simulink library "sm_rollerV_lib_terrain_contact_belem"  (R2026a)
settings: Solver=VariableStepAuto
undefined symbols (not defined in the file): Excv, L1, L2, L3, L4, L5, L6, L7, L8, L9, S1, S2, Scene, X, Y, Z
libraries: sm_lib x16, $bdroot x14, nesl_utility x10, sm_trackV_lib_terrain_contact_elem x6
Description:
  | Copyright 2024-2026 The MathWorks, Inc.
settings Model: Creator=smiller  LastModifiedBy=smiller

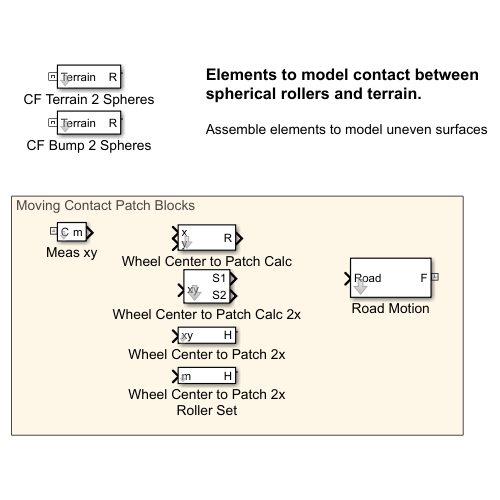
[thumbnail: Simulink's stored preview of the top-level diagram]
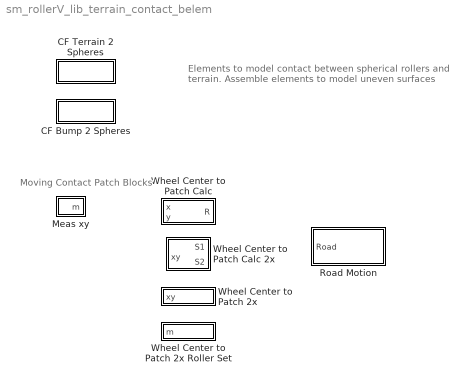
== system sm_rollerV_lib_terrain_contact_belem ==
  note: Moving Contact Patch Blocks
  note: Elements to model contact between
      | spherical rollers and terrain.
      |
      | Assemble elements to model uneven surfaces
  CF Bump 2 Spheres : Subsystem  mask(Contact Force, Two Spheres to Bump){K_BrickBump=Scene.Contact.BrickBump.K, B_BrickBump=Scene.Contact.BrickBump.B, TW_BrickBump=Scene.Contact.BrickBump.TW, CoefficientOfDynamicFriction=Scene.Contact.Terrain.mud, CoefficientOfStaticFriction=Scene.Contact.Terrain.mus, FrictionalCriticalVelocity=Scene.Contact.Terrain.CV}
      mask prompts: K_BrickBump "Normal Stiffness (N/m)"; B_BrickBump "Normal Damping (N/(m/s))"; TW_BrickBump "Normal Transition Width (m)"; CoefficientOfDynamicFriction "Coefficient of Dynamic Friction"; CoefficientOfStaticFriction "Coefficient of Static Friction"; FrictionalCriticalVelocity "Critical Velocity (m/s)"
      mask help: Models contact force between two spheres and a bump.
      mask TypeOptions K_BrickBump: CF Bump Roller Sphere 1 /NormalStiffness | CF Bump Roller Sphere 2/NormalStiffness
      mask TypeOptions B_BrickBump: CF Bump Roller Sphere 1 /NormalDamping | CF Bump Roller Sphere 2/NormalDamping
      mask TypeOptions TW_BrickBump: CF Bump Roller Sphere 1 /NormalTransitionRegionWidth | CF Bump Roller Sphere 2/NormalTransitionRegionWidth
      mask TypeOptions CoefficientOfDynamicFriction: CF Bump Roller Sphere 1 /CoefficientOfDynamicFriction | CF Bump Roller Sphere 2/CoefficientOfDynamicFriction
      mask TypeOptions CoefficientOfStaticFriction: CF Bump Roller Sphere 1 /CoefficientOfStaticFriction | CF Bump Roller Sphere 2/CoefficientOfStaticFriction
      mask TypeOptions FrictionalCriticalVelocity: CF Bump Roller Sphere 1 /FrictionalCriticalVelocity | CF Bump Roller Sphere 2/FrictionalCriticalVelocity
  CF Terrain 2 Spheres : Subsystem  mask(Contact Force, Two Spheres to Ground){NormalStiffness=Scene.Contact.Spheres.Terrain.K, NormalDamping=Scene.Contact.Spheres.Terrain.B, NormalTransitionRegionWidth=Scene.Contact.Spheres.Terrain.TW, CoefficientOfDynamicFriction=Scene.Contact.Spheres.Terrain.mud, CoefficientOfStaticFriction=Scene.Contact.Spheres.Terrain.mus, FrictionalCriticalVelocity=Scene.Contact.Spheres.Terrain.CV}
      mask prompts: NormalStiffness "Normal Stiffness (N/m)"; NormalDamping "Normal Damping (N/(m/s))"; NormalTransitionRegionWidth "Normal Transition Width (m)"; CoefficientOfDynamicFriction "Coefficient of Dynamic Friction"; CoefficientOfStaticFriction "Coefficient of Static Friction"; FrictionalCriticalVelocity "Critical Velocity (m/s)"
      mask help: Models contact force between two spheres and the ground.
      mask TypeOptions NormalStiffness: CF Roller Sphere Terrain 1/NormalStiffness | CF Roller Sphere Terrain 2/NormalStiffness
      mask TypeOptions NormalDamping: CF Roller Sphere Terrain 1/NormalDamping | CF Roller Sphere Terrain 2/NormalDamping
      mask TypeOptions NormalTransitionRegionWidth: CF Roller Sphere Terrain 1/NormalTransitionRegionWidth | CF Roller Sphere Terrain 2/NormalTransitionRegionWidth
      mask TypeOptions CoefficientOfDynamicFriction: CF Roller Sphere Terrain 1/CoefficientOfDynamicFriction | CF Roller Sphere Terrain 2/CoefficientOfDynamicFriction
      mask TypeOptions CoefficientOfStaticFriction: CF Roller Sphere Terrain 1/CoefficientOfStaticFriction | CF Roller Sphere Terrain 2/CoefficientOfStaticFriction
      mask TypeOptions FrictionalCriticalVelocity: CF Roller Sphere Terrain 1/FrictionalCriticalVelocity | CF Roller Sphere Terrain 2/FrictionalCriticalVelocity
  Meas xy : Subsystem  mask(Measure Cartesian Location of two frames){whl_offset=Excv.Shoe.w}
      mask prompts: whl_offset "Frame Offset"
      mask help: Measure position of two frames. Frames are separated by a distance along their common z-axis.
  Road Motion : Subsystem  mask(Position Infinite Plane){}
      mask help: Positions and orients Infinite Plane based on input signal. Abstract method of modeling objects contacting uneven terrain.
  Wheel Center to Patch 2x : Subsystem  mask(Wheel Center to Patch Height and Pitch, Infinite Planes){road_pz_x=Scene.Plateau.Road.pzLUT.px, road_pz_z=Scene.Plateau.Road.pzLUT.pz(:,1), road_qy_x=Scene.Plateau.Road.qyLUT.px, road_qy_qy=Scene.Plateau.Road.qyLUT.qy(:,1), tfilter=0.01, patch_clr=[0.5 0.5 0.5], patch_opc=0.25, patch_x=1, patch_y=1, NormalStiffness=Scene.Contact.Terrain.K, NormalDamping=Scene.Contact.Terrain.B, NormalTransitionRegionWidth=Scene.Contact.Terrain.TW, CoefficientOfDynamicFriction=Scene.Contact.Terrain.mud, CoefficientOfStaticFriction=Scene.Contact.Terrain.mus, FrictionalCriticalVelocity=Scene.Contact.Terrain.CV}
      mask prompts: road_pz_x "Road Distances (m)"; road_pz_z "Road Heights (m)"; road_qy_x "Road Distances(m)"; road_qy_qy "Road Pitch (m)"; tfilter "Filter Constant (seconds)"; patch_clr "Color [R G B] (0-1)"; patch_opc "Opacity (0-1)"; patch_x "Patch Length x (m)"; patch_y "Patch Length y (m)"; NormalStiffness "Normal Stiffness (N/m)"; NormalDamping "Normal Damping (N/(m/s))"; NormalTransitionRegionWidth "Normal Transition Width (m)"; CoefficientOfDynamicFriction "Coefficient of Dynamic Friction"; CoefficientOfStaticFriction "Coefficient of Static Friction"; FrictionalCriticalVelocity "Critical Velocity (m/s)"
      mask help: Find contact patch height and pitch using a lookup table, where the inputs are the x-y location of two frames. The output is a Simscape Bus with the geometry ports for Infinite Planes positioned and pitched for the two input frame locations.
      mask TypeOptions road_pz_x:
      | Wheel Center
      | to Patch/road_pz_x
      mask TypeOptions road_pz_z:
      | Wheel Center
      | to Patch/road_pz_z
      mask TypeOptions road_qy_x:
      | Wheel Center
      | to Patch/road_qy_x
      mask TypeOptions road_qy_qy:
      | Wheel Center
      | to Patch/road_qy_qy
      mask TypeOptions tfilter:
      | Wheel Center
      | to Patch/tfilter
      mask TypeOptions patch_clr: Infinite Plane1/GraphicDiffuseColor | Infinite Plane2/GraphicDiffuseColor
      mask TypeOptions patch_opc: Infinite Plane1/GraphicOpacity | Infinite Plane2/GraphicOpacity
      mask TypeOptions patch_x: Infinite Plane1/GraphicPlaneWidth | Infinite Plane2/GraphicPlaneWidth
      mask TypeOptions patch_y: Infinite Plane1/GraphicPlaneHeight | Infinite Plane2/GraphicPlaneHeight
      mask TypeOptions NormalStiffness: CF Track Terrain1/NormalStiffness | CF Track Terrain2/NormalStiffness
      mask TypeOptions NormalDamping: CF Track Terrain1/NormalDamping | CF Track Terrain2/NormalDamping
      mask TypeOptions NormalTransitionRegionWidth: CF Track Terrain1/NormalTransitionRegionWidth | CF Track Terrain2/NormalTransitionRegionWidth
      mask TypeOptions CoefficientOfDynamicFriction: CF Track Terrain1/CoefficientOfDynamicFriction | CF Track Terrain2/CoefficientOfDynamicFriction
      mask TypeOptions CoefficientOfStaticFriction: CF Track Terrain1/CoefficientOfStaticFriction | CF Track Terrain2/CoefficientOfStaticFriction
      mask TypeOptions FrictionalCriticalVelocity: CF Track Terrain1/FrictionalCriticalVelocity | CF Track Terrain2/FrictionalCriticalVelocity
      mask DialogControl cont_surface Prompt: Surface
      mask DialogControl cont_patchvis Prompt: Patch Visual
      mask DialogControl cont_contact Prompt: Contact
  Wheel Center to Patch 2x Roller Set : Subsystem  mask(Wheel Center to Patch Height and Pitch, All Rollers){road_pz_x=Scene.Plateau.Road.pzLUT.px, road_pz_z=Scene.Plateau.Road.pzLUT.pz(:,1), road_qy_x=Scene.Plateau.Road.qyLUT.px, road_qy_qy=Scene.Plateau.Road.qyLUT.qy(:,1), tfilter=0.01, NormalStiffness=Scene.Contact.Terrain.K, NormalDamping=Scene.Contact.Terrain.B, NormalTransitionRegionWidth=Scene.Contact.Terrain.TW, CoefficientOfDynamicFriction=Scene.Contact.Terrain.mud, CoefficientOfStaticFriction=Scene.Contact.Terrain.mus, FrictionalCriticalVelocity=Scene.Contact.Terrain.CV, patch_x=1, patch_y=1, patch_clr=[0.5 0.5 0.5], patch_opc=0.25}
      mask prompts: road_pz_x "Road Distances (m)"; road_pz_z "Road Heights (m)"; road_qy_x "Road Distances(m)"; road_qy_qy "Road Pitch (m)"; tfilter "Filter Constant (seconds)"; NormalStiffness "Normal Stiffness (N/m)"; NormalDamping "Normal Damping (N/(m/s))"; NormalTransitionRegionWidth "Normal Transition Width (m)"; CoefficientOfDynamicFriction "Coefficient of Dynamic Friction"; CoefficientOfStaticFriction "Coefficient of Static Friction"; FrictionalCriticalVelocity "Critical Velocity (m/s)"; patch_x "Patch Length x (m)"; patch_y "Patch Length y (m)"; patch_clr "Color [R G B] (0-1)"; patch_opc "Opacity (0-1)"
      mask help: Find contact patch height and pitch using a lookup table, where the inputs are the x-y location of two frames. The output is a Simscape Bus with the geometry ports for Infinite Planes positioned and pitched for all input frame locations.
      mask TypeOptions road_pz_x: Wheel Center to Patch Contact 1/road_pz_x | Wheel Center to Patch Contact 2/road_pz_x | Wheel Center to Patch Contact 3/road_pz_x | Wheel Center to Patch Contact 4/road_pz_x | Wheel Center to Patch Contact 5/road_pz_x | Wheel Center to Patch Contact 6/road_pz_x | Wheel Center to Patch Contact 7/road_pz_x | Wheel Center to Patch Contact 8/road_pz_x | Wheel Center to Patch Contact 9/road_pz_x
      mask TypeOptions road_pz_z: Wheel Center to Patch Contact 1/road_pz_z | Wheel Center to Patch Contact 2/road_pz_z | Wheel Center to Patch Contact 3/road_pz_z | Wheel Center to Patch Contact 4/road_pz_z | Wheel Center to Patch Contact 5/road_pz_z | Wheel Center to Patch Contact 6/road_pz_z | Wheel Center to Patch Contact 7/road_pz_z | Wheel Center to Patch Contact 8/road_pz_z | Wheel Center to Patch Contact 9/road_pz_z
      mask TypeOptions road_qy_x: Wheel Center to Patch Contact 1/road_qy_x | Wheel Center to Patch Contact 2/road_qy_x | Wheel Center to Patch Contact 3/road_qy_x | Wheel Center to Patch Contact 4/road_qy_x | Wheel Center to Patch Contact 5/road_qy_x | Wheel Center to Patch Contact 6/road_qy_x | Wheel Center to Patch Contact 7/road_qy_x | Wheel Center to Patch Contact 8/road_qy_x | Wheel Center to Patch Contact 9/road_qy_x
      mask TypeOptions road_qy_qy: Wheel Center to Patch Contact 1/road_qy_qy | Wheel Center to Patch Contact 2/road_qy_qy | Wheel Center to Patch Contact 3/road_qy_qy | Wheel Center to Patch Contact 4/road_qy_qy | Wheel Center to Patch Contact 5/road_qy_qy | Wheel Center to Patch Contact 6/road_qy_qy | Wheel Center to Patch Contact 7/road_qy_qy | Wheel Center to Patch Contact 8/road_qy_qy | Wheel Center to Patch Contact 9/road_qy_qy
      mask TypeOptions tfilter: Wheel Center to Patch Contact 1/tfilter | Wheel Center to Patch Contact 2/tfilter | Wheel Center to Patch Contact 3/tfilter | Wheel Center to Patch Contact 4/tfilter | Wheel Center to Patch Contact 5/tfilter | Wheel Center to Patch Contact 6/tfilter | Wheel Center to Patch Contact 7/tfilter | Wheel Center to Patch Contact 8/tfilter | Wheel Center to Patch Contact 9/tfilter
      mask TypeOptions NormalStiffness: Wheel Center to Patch Contact 1/NormalStiffness | Wheel Center to Patch Contact 2/NormalStiffness | Wheel Center to Patch Contact 3/NormalStiffness | Wheel Center to Patch Contact 4/NormalStiffness | Wheel Center to Patch Contact 5/NormalStiffness | Wheel Center to Patch Contact 6/NormalStiffness | Wheel Center to Patch Contact 7/NormalStiffness | Wheel Center to Patch Contact 8/NormalStiffness | Wheel Center to Patch Contact 9/NormalStiffness
      mask TypeOptions NormalDamping: Wheel Center to Patch Contact 1/NormalDamping | Wheel Center to Patch Contact 2/NormalDamping | Wheel Center to Patch Contact 3/NormalDamping | Wheel Center to Patch Contact 4/NormalDamping | Wheel Center to Patch Contact 5/NormalDamping | Wheel Center to Patch Contact 6/NormalDamping | Wheel Center to Patch Contact 7/NormalDamping | Wheel Center to Patch Contact 8/NormalDamping | Wheel Center to Patch Contact 9/NormalDamping
      mask TypeOptions NormalTransitionRegionWidth: Wheel Center to Patch Contact 1/NormalTransitionRegionWidth | Wheel Center to Patch Contact 2/NormalTransitionRegionWidth | Wheel Center to Patch Contact 3/NormalTransitionRegionWidth | Wheel Center to Patch Contact 4/NormalTransitionRegionWidth | Wheel Center to Patch Contact 5/NormalTransitionRegionWidth | Wheel Center to Patch Contact 6/NormalTransitionRegionWidth | Wheel Center to Patch Contact 7/NormalTransitionRegionWidth | Wheel Center to Patch Contact 8/NormalTransitionRegionWidth | Wheel Center to Patch Contact 9/NormalTransitionRegionWidth
      mask TypeOptions CoefficientOfDynamicFriction: Wheel Center to Patch Contact 1/CoefficientOfDynamicFriction | Wheel Center to Patch Contact 2/CoefficientOfDynamicFriction | Wheel Center to Patch Contact 3/CoefficientOfDynamicFriction | Wheel Center to Patch Contact 4/CoefficientOfDynamicFriction | Wheel Center to Patch Contact 5/CoefficientOfDynamicFriction | Wheel Center to Patch Contact 6/CoefficientOfDynamicFriction | Wheel Center to Patch Contact 7/CoefficientOfDynamicFriction | Wheel Center to Patch Contact 8/CoefficientOfDynamicFriction | Wheel Center to Patch Contact 9/CoefficientOfDynamicFriction
      mask TypeOptions CoefficientOfStaticFriction: Wheel Center to Patch Contact 1/CoefficientOfStaticFriction | Wheel Center to Patch Contact 2/CoefficientOfStaticFriction | Wheel Center to Patch Contact 3/CoefficientOfStaticFriction | Wheel Center to Patch Contact 4/CoefficientOfStaticFriction | Wheel Center to Patch Contact 5/CoefficientOfStaticFriction | Wheel Center to Patch Contact 6/CoefficientOfStaticFriction | Wheel Center to Patch Contact 7/CoefficientOfStaticFriction | Wheel Center to Patch Contact 8/CoefficientOfStaticFriction | Wheel Center to Patch Contact 9/CoefficientOfStaticFriction
      mask TypeOptions FrictionalCriticalVelocity: Wheel Center to Patch Contact 1/FrictionalCriticalVelocity | Wheel Center to Patch Contact 2/FrictionalCriticalVelocity | Wheel Center to Patch Contact 3/FrictionalCriticalVelocity | Wheel Center to Patch Contact 4/FrictionalCriticalVelocity | Wheel Center to Patch Contact 5/FrictionalCriticalVelocity | Wheel Center to Patch Contact 6/FrictionalCriticalVelocity | Wheel Center to Patch Contact 7/FrictionalCriticalVelocity | Wheel Center to Patch Contact 8/FrictionalCriticalVelocity | Wheel Center to Patch Contact 9/FrictionalCriticalVelocity
      mask TypeOptions patch_x: Wheel Center to Patch Contact 1/patch_x | Wheel Center to Patch Contact 2/patch_x | Wheel Center to Patch Contact 3/patch_x | Wheel Center to Patch Contact 4/patch_x | Wheel Center to Patch Contact 5/patch_x | Wheel Center to Patch Contact 6/patch_x | Wheel Center to Patch Contact 7/patch_x | Wheel Center to Patch Contact 8/patch_x | Wheel Center to Patch Contact 9/patch_x
      mask TypeOptions patch_y: Wheel Center to Patch Contact 1/patch_y | Wheel Center to Patch Contact 2/patch_y | Wheel Center to Patch Contact 3/patch_y | Wheel Center to Patch Contact 4/patch_y | Wheel Center to Patch Contact 5/patch_y | Wheel Center to Patch Contact 6/patch_y | Wheel Center to Patch Contact 7/patch_y | Wheel Center to Patch Contact 8/patch_y | Wheel Center to Patch Contact 9/patch_y
      mask TypeOptions patch_clr: Wheel Center to Patch Contact 1/patch_clr | Wheel Center to Patch Contact 2/patch_clr | Wheel Center to Patch Contact 3/patch_clr | Wheel Center to Patch Contact 4/patch_clr | Wheel Center to Patch Contact 5/patch_clr | Wheel Center to Patch Contact 6/patch_clr | Wheel Center to Patch Contact 7/patch_clr | Wheel Center to Patch Contact 8/patch_clr | Wheel Center to Patch Contact 9/patch_clr
      mask TypeOptions patch_opc: Wheel Center to Patch Contact 1/patch_opc | Wheel Center to Patch Contact 2/patch_opc | Wheel Center to Patch Contact 3/patch_opc | Wheel Center to Patch Contact 4/patch_opc | Wheel Center to Patch Contact 5/patch_opc | Wheel Center to Patch Contact 6/patch_opc | Wheel Center to Patch Contact 7/patch_opc | Wheel Center to Patch Contact 8/patch_opc | Wheel Center to Patch Contact 9/patch_opc
      mask DialogControl cont_surface Prompt: Surface
      mask DialogControl cont_surfHeight Prompt: Height
      mask DialogControl cont_surfPitch Prompt: Pitch
      mask DialogControl cont_contact Prompt: Contact
      mask DialogControl cont_patchvis Prompt: Patch Visual
  Wheel Center to Patch Calc : Subsystem  mask(Wheel Center to Patch Height and Pitch){road_pz_x=Scene.Plateau.Road.pzLUT.px, road_pz_z=Scene.Plateau.Road.pzLUT.pz(:,1), road_qy_x=Scene.Plateau.Road.qyLUT.px, road_qy_qy=Scene.Plateau.Road.qyLUT.qy(:,1)}
      mask prompts: road_pz_x "Road Distances (m)"; road_pz_z "Road Heights (m)"; road_qy_x "Road Distances(m)"; road_qy_qy "Road Pitch (m)"
      mask help: Find contact patch height and pitch using a lookup table, where the inputs are the x-y location of the frame.
      mask DialogControl cont_roadpz Prompt: Road Height
      mask DialogControl cont_roadqy Prompt: Road Pitch
  Wheel Center to Patch Calc 2x : Subsystem  mask(Wheel Center to Patch Height and Pitch, Two Frames){road_pz_x=Scene.Plateau.Road.pzLUT.px, road_pz_z=Scene.Plateau.Road.pzLUT.pz(:,1), road_qy_x=Scene.Plateau.Road.qyLUT.px, road_qy_qy=Scene.Plateau.Road.qyLUT.qy(:,1), tfilter=0.01}
      mask prompts: road_pz_x "Road Distances (m)"; road_pz_z "Road Heights (m)"; road_qy_x "Road Distances(m)"; road_qy_qy "Road Pitch (m)"; tfilter "Filter Constant (seconds)"
      mask help: Find contact patch height and pitch using a lookup table, where the inputs are the x-y location of two frames.
      mask TypeOptions road_pz_x: Wheel Center to Patch1/road_pz_x | Wheel Center to Patch2/road_pz_x
      mask TypeOptions road_pz_z: Wheel Center to Patch1/road_pz_z | Wheel Center to Patch2/road_pz_z
      mask TypeOptions road_qy_x: Wheel Center to Patch1/road_qy_x | Wheel Center to Patch2/road_qy_x
      mask TypeOptions road_qy_qy: Wheel Center to Patch1/road_qy_qy | Wheel Center to Patch2/road_qy_qy

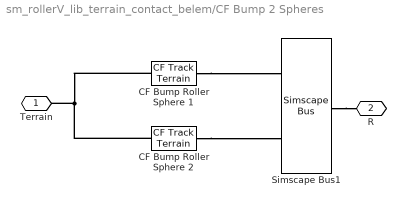
== system sm_rollerV_lib_terrain_contact_belem/CF Bump 2 Spheres ==
  "CF Bump Roller Sphere 1 " : sm_trackV_lib_terrain_contact_elem/CF Track Terrain  NormalStiffness=K_BrickBump  NormalDamping=B_BrickBump  NormalTransitionRegionWidth=TW_BrickBump  CoefficientOfDynamicFriction=CoefficientOfDynamicFriction  CoefficientOfStaticFriction=CoefficientOfStaticFriction  FrictionalCriticalVelocity=FrictionalCriticalVelocity
  CF Bump Roller Sphere 2 : sm_trackV_lib_terrain_contact_elem/CF Track Terrain  NormalStiffness=K_BrickBump  NormalDamping=B_BrickBump  NormalTransitionRegionWidth=TW_BrickBump  CoefficientOfDynamicFriction=CoefficientOfDynamicFriction  CoefficientOfStaticFriction=CoefficientOfStaticFriction  FrictionalCriticalVelocity=FrictionalCriticalVelocity
  Simscape Bus1 : SimscapeBus  HierarchyStrings=S1;S2
  Terrain : PMIOPort  Side=Left
  R : PMIOPort  Port=2  Side=Right
  connections:
  "CF Bump Roller Sphere 1 "/RConn1 -- Simscape Bus1/LConn1
  "CF Bump Roller Sphere 1 "/LConn1 -- CF Bump Roller Sphere 2/LConn1 -- Terrain/RConn1
  CF Bump Roller Sphere 2/RConn1 -- Simscape Bus1/LConn2
  Simscape Bus1/RConn1 -- R/RConn1

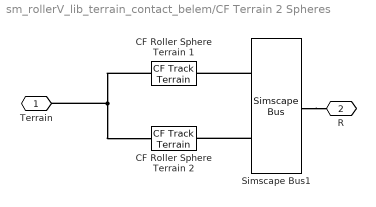
== system sm_rollerV_lib_terrain_contact_belem/CF Terrain 2 Spheres ==
  CF Roller Sphere Terrain 1 : sm_trackV_lib_terrain_contact_elem/CF Track Terrain  NormalStiffness=NormalStiffness  NormalDamping=NormalDamping  NormalTransitionRegionWidth=NormalTransitionRegionWidth  CoefficientOfDynamicFriction=CoefficientOfDynamicFriction  CoefficientOfStaticFriction=CoefficientOfStaticFriction  FrictionalCriticalVelocity=FrictionalCriticalVelocity
  CF Roller Sphere Terrain 2 : sm_trackV_lib_terrain_contact_elem/CF Track Terrain  NormalStiffness=NormalStiffness  NormalDamping=NormalDamping  NormalTransitionRegionWidth=NormalTransitionRegionWidth  CoefficientOfDynamicFriction=CoefficientOfDynamicFriction  CoefficientOfStaticFriction=CoefficientOfStaticFriction  FrictionalCriticalVelocity=FrictionalCriticalVelocity
  Simscape Bus1 : SimscapeBus  HierarchyStrings=S1;S2
  Terrain : PMIOPort  Side=Left
  R : PMIOPort  Port=2  Side=Right
  connections:
  Simscape Bus1/RConn1 -- R/RConn1
  Simscape Bus1/LConn2 -- CF Roller Sphere Terrain 2/RConn1
  Terrain/RConn1 -- CF Roller Sphere Terrain 2/LConn1 -- CF Roller Sphere Terrain 1/LConn1
  Simscape Bus1/LConn1 -- CF Roller Sphere Terrain 1/RConn1

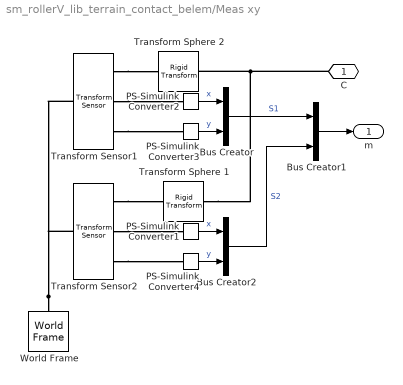
== system sm_rollerV_lib_terrain_contact_belem/Meas xy ==
  Bus Creator : BusCreator  Inputs=2
  Bus Creator1 : BusCreator  Inputs=2
  Bus Creator2 : BusCreator  Inputs=2
  PS-Simulink Converter{1..4} (4 alike) : nesl_utility/PS-Simulink Converter  PhysicalDomain=network_engine_domain  SubClassName=ps_output  LeftPortType=input  RightPortType=output  PseudoPeriodic=off  Frequencies=[]  VectorFormat=inherit  Unit=inherit  AffineConversion=off
  Transform Sensor1 : sm_lib/Frames and Transforms/Transform Sensor  MeasurementFrame=World  RotationSequence=XYX  SenseAngle=off  SenseAxis=off  SenseQ=off  SenseR=off  SenseRotationSequence=off  SenseOmegaX=off  SenseOmegaY=off  SenseOmegaZ=off  SenseOmega=off  SenseQDot=off  SenseRDot=off  SenseRotationSequenceDot=off  SenseAlphaX=off  SenseAlphaY=off  SenseAlphaZ=off  SenseAlpha=off  SenseQDDot=off  SenseRDDot=off  SenseX=on  SenseY=on  SenseZ=off  SenseXYZ=off  SenseRad=off  SenseAzim=off  SenseDist=off  SenseInc=off  SenseXDot=off  SenseYDot=off  SenseZDot=off  SenseXYZDot=off  SenseRadDot=off  SenseAzimDot=off  SenseDistDot=off  SenseIncDot=off  SenseXDDot=off  SenseYDDot=off  SenseZDDot=off  SenseXYZDDot=off  SenseRadDDot=off  SenseAzimDDot=off  SenseDistDDot=off  SenseIncDDot=off
  Transform Sensor2 : sm_lib/Frames and Transforms/Transform Sensor  MeasurementFrame=World  RotationSequence=XYX  SenseAngle=off  SenseAxis=off  SenseQ=off  SenseR=off  SenseRotationSequence=off  SenseOmegaX=off  SenseOmegaY=off  SenseOmegaZ=off  SenseOmega=off  SenseQDot=off  SenseRDot=off  SenseRotationSequenceDot=off  SenseAlphaX=off  SenseAlphaY=off  SenseAlphaZ=off  SenseAlpha=off  SenseQDDot=off  SenseRDDot=off  SenseX=on  SenseY=on  SenseZ=off  SenseXYZ=off  SenseRad=off  SenseAzim=off  SenseDist=off  SenseInc=off  SenseXDot=off  SenseYDot=off  SenseZDot=off  SenseXYZDot=off  SenseRadDot=off  SenseAzimDot=off  SenseDistDot=off  SenseIncDot=off  SenseXDDot=off  SenseYDDot=off  SenseZDDot=off  SenseXYZDDot=off  SenseRadDDot=off  SenseAzimDDot=off  SenseDistDDot=off  SenseIncDDot=off
  Transform Sphere 1 : sm_lib/Frames and Transforms/Rigid Transform  RotationMethod=None  FollAlignAxisA=+X  BaseAlignAxisA=+Y  FollAlignAxisB=+Y  BaseAlignAxisB=+Z  RotationStandardAxis=+Z  RotationAngle=0.0  RotationAngleUnits=deg  RotationArbitraryAxis=[0 0 1]  RotationSequenceAxes=FollowerAxes  RotationSequence=XYX  RotationSequenceAngles=[0 0 0]  RotationSequenceAnglesUnits=deg  RotationMatrix=[1 0 0; 0 1 0; 0 0 1]  Quaternion=[1 0 0 0]  TranslationMethod=StandardAxis  TranslationCartesianOffset=[0 0 0]  TranslationCartesianOffsetUnits=m  TranslationStandardAxis=+Z  TranslationStandardOffset=whl_offset/2  TranslationStandardOffsetUnits=m  TranslationROffset=0  TranslationROffsetUnits=m  TranslationThetaOffset=0  TranslationThetaOffsetUnits=deg  TranslationZOffset=0  TranslationZOffsetUnits=m
  Transform Sphere 2 : sm_lib/Frames and Transforms/Rigid Transform  RotationMethod=None  FollAlignAxisA=+X  BaseAlignAxisA=+Y  FollAlignAxisB=+Y  BaseAlignAxisB=+Z  RotationStandardAxis=+Z  RotationAngle=0.0  RotationAngleUnits=deg  RotationArbitraryAxis=[0 0 1]  RotationSequenceAxes=FollowerAxes  RotationSequence=XYX  RotationSequenceAngles=[0 0 0]  RotationSequenceAnglesUnits=deg  RotationMatrix=[1 0 0; 0 1 0; 0 0 1]  Quaternion=[1 0 0 0]  TranslationMethod=StandardAxis  TranslationCartesianOffset=[0 0 0]  TranslationCartesianOffsetUnits=m  TranslationStandardAxis=+Z  TranslationStandardOffset=-whl_offset/2  TranslationStandardOffsetUnits=m  TranslationROffset=0  TranslationROffsetUnits=m  TranslationThetaOffset=0  TranslationThetaOffsetUnits=deg  TranslationZOffset=0  TranslationZOffsetUnits=m
  World Frame : sm_lib/Frames and Transforms/World Frame
  C : PMIOPort  Side=Left
  m : Outport
  wires:
  PS-Simulink Converter3/1 -> Bus Creator/2  "y"
  PS-Simulink Converter2/1 -> Bus Creator/1  "x"
  Bus Creator/1 -> Bus Creator1/1  "S1"
  Bus Creator1/1 -> m/1
  Bus Creator2/1 -> Bus Creator1/2  "S2"
  PS-Simulink Converter1/1 -> Bus Creator2/1  "x"
  PS-Simulink Converter4/1 -> Bus Creator2/2  "y"
  connections:
  World Frame/RConn1 -- Transform Sensor1/LConn1 -- Transform Sensor2/LConn1
  Transform Sensor1/RConn3 -- PS-Simulink Converter3/LConn1
  Transform Sensor1/RConn1 -- Transform Sphere 2/RConn1
  Transform Sensor1/RConn2 -- PS-Simulink Converter2/LConn1
  Transform Sphere 1/LConn1 -- C/RConn1 -- Transform Sphere 2/LConn1
  Transform Sensor2/RConn2 -- PS-Simulink Converter1/LConn1
  Transform Sensor2/RConn3 -- PS-Simulink Converter4/LConn1
  Transform Sensor2/RConn1 -- Transform Sphere 1/RConn1

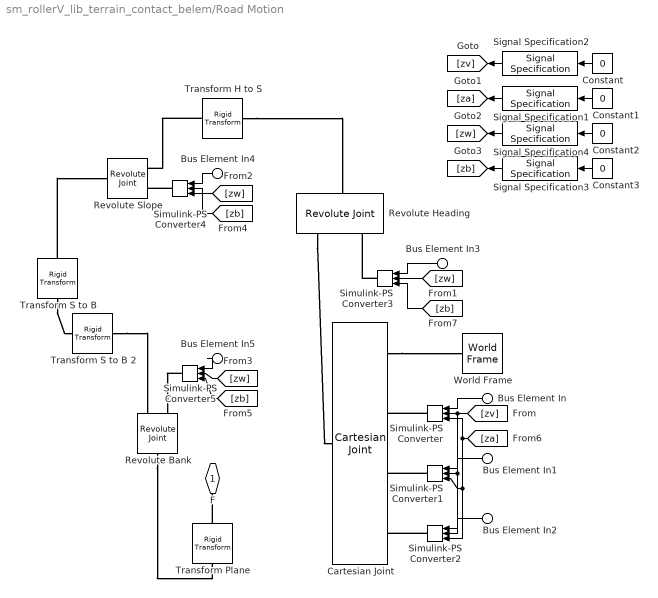
== system sm_rollerV_lib_terrain_contact_belem/Road Motion ==
  Bus Element In : Inport  PortName=Road  Element=px
  Bus Element In1 : Inport  PortName=Road  Element=py
  Bus Element In2 : Inport  PortName=Road  Element=pz
  Bus Element In3 : Inport  PortName=Road  Element=qz
  Bus Element In4 : Inport  PortName=Road  Element=qy
  Bus Element In5 : Inport  PortName=Road  Element=qx
  Cartesian Joint : sm_lib/Joints/Cartesian Joint  JointMode=Normal  CompositeWrenchDir=FollowerOnBase  CompositeWrenchFrame=BaseFrame  SenseConstraintForce=off  SenseConstraintTorque=off  SenseTotalForce=off  SenseTotalTorque=off  PxPositionTargetSpecify=off  PxPositionTargetPriority=High  PxPositionTargetValue=0  PxPositionTargetValueUnits=m  PxVelocityTargetSpecify=off  PxVelocityTargetPriority=High  PxVelocityTargetValue=0  PxVelocityTargetValueUnits=m/s  PxEquilibriumPosition=0  PxEquilibriumPositionUnits=m  PxSpringStiffness=0  PxSpringStiffnessUnits=N/m  PxDampingCoefficient=0  PxDampingCoefficientUnits=N/(m/s)  PxLowerLimitSpecify=off  PxLowerLimitBound=-1  PxLowerLimitBoundUnits=m  PxLowerLimitStiffness=1e6  PxLowerLimitStiffnessUnits=N/m  PxLowerLimitDamping=1e3  PxLowerLimitDampingUnits=N/(m/s)  PxLowerLimitTransitionRegionWidth=1e-4  PxLowerLimitTransitionRegionWidthUnits=m  PxUpperLimitSpecify=off  PxUpperLimitBound=1  PxUpperLimitBoundUnits=m  PxUpperLimitStiffness=1e6  PxUpperLimitStiffnessUnits=N/m  PxUpperLimitDamping=1e3  PxUpperLimitDampingUnits=N/(m/s)  PxUpperLimitTransitionRegionWidth=1e-4  PxUpperLimitTransitionRegionWidthUnits=m  PxTorqueActuationMode=ComputedTorque  PxMotionActuationMode=InputMotion  PxSensePosition=off  PxSenseVelocity=off  PxSenseAcceleration=off  PxSenseTorqueForce=off  PxSenseLowerLimitTorqueForce=off  PxSenseUpperLimitTorqueForce=off  PyPositionTargetSpecify=off  PyPositionTargetPriority=High  PyPositionTargetValue=0  PyPositionTargetValueUnits=m  PyVelocityTargetSpecify=off  PyVelocityTargetPriority=High  PyVelocityTargetValue=0  PyVelocityTargetValueUnits=m/s  PyEquilibriumPosition=0  PyEquilibriumPositionUnits=m  PySpringStiffness=0  PySpringStiffnessUnits=N/m  PyDampingCoefficient=0  PyDampingCoefficientUnits=N/(m/s)  PyLowerLimitSpecify=off  PyLowerLimitBound=-1  PyLowerLimitBoundUnits=m  PyLowerLimitStiffness=1e6  PyLowerLimitStiffnessUnits=N/m  PyLowerLimitDamping=1e3  PyLowerLimitDampingUnits=N/(m/s)  PyLowerLimitTransitionRegionWidth=1e-4  PyLowerLimitTransitionRegionWidthUnits=m  PyUpperLimitSpecify=off  PyUpperLimitBound=1  PyUpperLimitBoundUnits=m  PyUpperLimitStiffness=1e6  PyUpperLimitStiffnessUnits=N/m  PyUpperLimitDamping=1e3  PyUpperLimitDampingUnits=N/(m/s)  PyUpperLimitTransitionRegionWidth=1e-4  PyUpperLimitTransitionRegionWidthUnits=m  PyTorqueActuationMode=ComputedTorque  PyMotionActuationMode=InputMotion  PySensePosition=off  PySenseVelocity=off  PySenseAcceleration=off  PySenseTorqueForce=off  PySenseLowerLimitTorqueForce=off  PySenseUpperLimitTorqueForce=off  PzPositionTargetSpecify=off  PzPositionTargetPriority=High  PzPositionTargetValue=0  PzPositionTargetValueUnits=m  PzVelocityTargetSpecify=off  PzVelocityTargetPriority=High  PzVelocityTargetValue=0  PzVelocityTargetValueUnits=m/s  PzEquilibriumPosition=0  PzEquilibriumPositionUnits=m  PzSpringStiffness=0  PzSpringStiffnessUnits=N/m  PzDampingCoefficient=0  PzDampingCoefficientUnits=N/(m/s)  PzLowerLimitSpecify=off  PzLowerLimitBound=-1  PzLowerLimitBoundUnits=m  PzLowerLimitStiffness=1e6  PzLowerLimitStiffnessUnits=N/m  PzLowerLimitDamping=1e3  PzLowerLimitDampingUnits=N/(m/s)  PzLowerLimitTransitionRegionWidth=1e-4  PzLowerLimitTransitionRegionWidthUnits=m  PzUpperLimitSpecify=off  PzUpperLimitBound=1  PzUpperLimitBoundUnits=m  PzUpperLimitStiffness=1e6  PzUpperLimitStiffnessUnits=N/m  PzUpperLimitDamping=1e3  PzUpperLimitDampingUnits=N/(m/s)  PzUpperLimitTransitionRegionWidth=1e-4  PzUpperLimitTransitionRegionWidthUnits=m  PzTorqueActuationMode=ComputedTorque  PzMotionActuationMode=InputMotion  PzSensePosition=off  PzSenseVelocity=off  PzSenseAcceleration=off  PzSenseTorqueForce=off  PzSenseLowerLimitTorqueForce=off  PzSenseUpperLimitTorqueForce=off
  Constant{,1..3} (4 alike) : Constant  Value=0
  Revolute Heading : sm_lib/Joints/Revolute Joint  JointMode=Normal  CompositeWrenchDir=FollowerOnBase  CompositeWrenchFrame=BaseFrame  SenseConstraintForce=off  SenseConstraintTorque=off  SenseTotalForce=off  SenseTotalTorque=off  PositionTargetSpecify=off  PositionTargetPriority=High  PositionTargetValue=0  PositionTargetValueUnits=deg  VelocityTargetSpecify=off  VelocityTargetPriority=High  VelocityTargetValue=0  VelocityTargetValueUnits=deg/s  EquilibriumPosition=0  EquilibriumPositionUnits=deg  SpringStiffness=0  SpringStiffnessUnits=N*m/deg  DampingCoefficient=0  DampingCoefficientUnits=N*m/(deg/s)  LowerLimitSpecify=off  LowerLimitBound=-90  LowerLimitBoundUnits=deg  LowerLimitStiffness=1e4  LowerLimitStiffnessUnits=N*m/deg  LowerLimitDamping=10  LowerLimitDampingUnits=N*m/(deg/s)  LowerLimitTransitionRegionWidth=0.1  LowerLimitTransitionRegionWidthUnits=deg  UpperLimitSpecify=off  UpperLimitBound=90  UpperLimitBoundUnits=deg  UpperLimitStiffness=1e4  UpperLimitStiffnessUnits=N*m/deg  UpperLimitDamping=10  UpperLimitDampingUnits=N*m/(deg/s)  UpperLimitTransitionRegionWidth=0.1  UpperLimitTransitionRegionWidthUnits=deg  TorqueActuationMode=ComputedTorque  MotionActuationMode=InputMotion  SensePosition=off  SenseVelocity=off  SenseAcceleration=off  SenseTorqueForce=off  SenseLowerLimitTorqueForce=off  SenseUpperLimitTorqueForce=off
  Revolute Slope : sm_lib/Joints/Revolute Joint  JointMode=Normal  CompositeWrenchDir=FollowerOnBase  CompositeWrenchFrame=BaseFrame  SenseConstraintForce=off  SenseConstraintTorque=off  SenseTotalForce=off  SenseTotalTorque=off  PositionTargetSpecify=off  PositionTargetPriority=High  PositionTargetValue=0  PositionTargetValueUnits=deg  VelocityTargetSpecify=off  VelocityTargetPriority=High  VelocityTargetValue=0  VelocityTargetValueUnits=deg/s  EquilibriumPosition=0  EquilibriumPositionUnits=deg  SpringStiffness=0  SpringStiffnessUnits=N*m/deg  DampingCoefficient=0  DampingCoefficientUnits=N*m/(deg/s)  LowerLimitSpecify=off  LowerLimitBound=-90  LowerLimitBoundUnits=deg  LowerLimitStiffness=1e4  LowerLimitStiffnessUnits=N*m/deg  LowerLimitDamping=10  LowerLimitDampingUnits=N*m/(deg/s)  LowerLimitTransitionRegionWidth=0.1  LowerLimitTransitionRegionWidthUnits=deg  UpperLimitSpecify=off  UpperLimitBound=90  UpperLimitBoundUnits=deg  UpperLimitStiffness=1e4  UpperLimitStiffnessUnits=N*m/deg  UpperLimitDamping=10  UpperLimitDampingUnits=N*m/(deg/s)  UpperLimitTransitionRegionWidth=0.1  UpperLimitTransitionRegionWidthUnits=deg  TorqueActuationMode=ComputedTorque  MotionActuationMode=InputMotion  SensePosition=off  SenseVelocity=off  SenseAcceleration=off  SenseTorqueForce=off  SenseLowerLimitTorqueForce=off  SenseUpperLimitTorqueForce=off
  Revolute Bank : sm_lib/Joints/Revolute Joint  JointMode=Normal  CompositeWrenchDir=FollowerOnBase  CompositeWrenchFrame=BaseFrame  SenseConstraintForce=off  SenseConstraintTorque=off  SenseTotalForce=off  SenseTotalTorque=off  PositionTargetSpecify=off  PositionTargetPriority=High  PositionTargetValue=0  PositionTargetValueUnits=deg  VelocityTargetSpecify=off  VelocityTargetPriority=High  VelocityTargetValue=0  VelocityTargetValueUnits=deg/s  EquilibriumPosition=0  EquilibriumPositionUnits=deg  SpringStiffness=0  SpringStiffnessUnits=N*m/deg  DampingCoefficient=0  DampingCoefficientUnits=N*m/(deg/s)  LowerLimitSpecify=off  LowerLimitBound=-90  LowerLimitBoundUnits=deg  LowerLimitStiffness=1e4  LowerLimitStiffnessUnits=N*m/deg  LowerLimitDamping=10  LowerLimitDampingUnits=N*m/(deg/s)  LowerLimitTransitionRegionWidth=0.1  LowerLimitTransitionRegionWidthUnits=deg  UpperLimitSpecify=off  UpperLimitBound=90  UpperLimitBoundUnits=deg  UpperLimitStiffness=1e4  UpperLimitStiffnessUnits=N*m/deg  UpperLimitDamping=10  UpperLimitDampingUnits=N*m/(deg/s)  UpperLimitTransitionRegionWidth=0.1  UpperLimitTransitionRegionWidthUnits=deg  TorqueActuationMode=ComputedTorque  MotionActuationMode=InputMotion  SensePosition=off  SenseVelocity=off  SenseAcceleration=off  SenseTorqueForce=off  SenseLowerLimitTorqueForce=off  SenseUpperLimitTorqueForce=off
  Signal Specification1 : SignalSpecification  Unit=m/s^2
  Signal Specification2 : SignalSpecification  Unit=m/s
  Signal Specification3 : SignalSpecification  Unit=rad/s^2
  Signal Specification4 : SignalSpecification  Unit=rad/s
  Simulink-PS Converter : nesl_utility/Simulink-PS Converter  PhysicalDomain=network_engine_domain  SubClassName=ps_input  LeftPortType=input  RightPortType=output  PseudoPeriodic=off  Frequencies=[]  NoiseDistribution=none  NoiseParameters=[]  Unit=m  AffineConversion=off  FilteringAndDerivatives=provide  SimscapeFilterOrder=1  InputFilterTimeConstant=0.001  UdotUserProvided=2
  Simulink-PS Converter1 : nesl_utility/Simulink-PS Converter  PhysicalDomain=network_engine_domain  SubClassName=ps_input  LeftPortType=input  RightPortType=output  PseudoPeriodic=off  Frequencies=[]  NoiseDistribution=none  NoiseParameters=[]  Unit=m  AffineConversion=off  FilteringAndDerivatives=provide  SimscapeFilterOrder=1  InputFilterTimeConstant=0.001  UdotUserProvided=2
  Simulink-PS Converter2 : nesl_utility/Simulink-PS Converter  PhysicalDomain=network_engine_domain  SubClassName=ps_input  LeftPortType=input  RightPortType=output  PseudoPeriodic=off  Frequencies=[]  NoiseDistribution=none  NoiseParameters=[]  Unit=m  AffineConversion=off  FilteringAndDerivatives=provide  SimscapeFilterOrder=1  InputFilterTimeConstant=0.001  UdotUserProvided=2
  Simulink-PS Converter3 : nesl_utility/Simulink-PS Converter  PhysicalDomain=network_engine_domain  SubClassName=ps_input  LeftPortType=input  RightPortType=output  PseudoPeriodic=off  Frequencies=[]  NoiseDistribution=none  NoiseParameters=[]  Unit=rad  AffineConversion=off  FilteringAndDerivatives=provide  SimscapeFilterOrder=1  InputFilterTimeConstant=0.001  UdotUserProvided=2
  Simulink-PS Converter4 : nesl_utility/Simulink-PS Converter  PhysicalDomain=network_engine_domain  SubClassName=ps_input  LeftPortType=input  RightPortType=output  PseudoPeriodic=off  Frequencies=[]  NoiseDistribution=none  NoiseParameters=[]  Unit=rad  AffineConversion=off  FilteringAndDerivatives=provide  SimscapeFilterOrder=1  InputFilterTimeConstant=0.001  UdotUserProvided=2
  Simulink-PS Converter5 : nesl_utility/Simulink-PS Converter  PhysicalDomain=network_engine_domain  SubClassName=ps_input  LeftPortType=input  RightPortType=output  PseudoPeriodic=off  Frequencies=[]  NoiseDistribution=none  NoiseParameters=[]  Unit=rad  AffineConversion=off  FilteringAndDerivatives=provide  SimscapeFilterOrder=1  InputFilterTimeConstant=0.001  UdotUserProvided=2
  Transform H to S : sm_lib/Frames and Transforms/Rigid Transform  RotationMethod=AlignedAxes  FollAlignAxisA=+Z  BaseAlignAxisA=+Y  FollAlignAxisB=+X  BaseAlignAxisB=+X  RotationStandardAxis=+Z  RotationAngle=0.0  RotationAngleUnits=deg  RotationArbitraryAxis=[0 0 1]  RotationSequenceAxes=FollowerAxes  RotationSequence=XYX  RotationSequenceAngles=[0 0 0]  RotationSequenceAnglesUnits=deg  RotationMatrix=[1 0 0; 0 1 0; 0 0 1]  Quaternion=[1 0 0 0]  TranslationMethod=None  TranslationCartesianOffset=[0 0 0]  TranslationCartesianOffsetUnits=m  TranslationStandardAxis=+Z  TranslationStandardOffset=0  TranslationStandardOffsetUnits=m  TranslationROffset=0  TranslationROffsetUnits=m  TranslationThetaOffset=0  TranslationThetaOffsetUnits=deg  TranslationZOffset=0  TranslationZOffsetUnits=m
  Transform Plane : sm_lib/Frames and Transforms/Rigid Transform  RotationMethod=AlignedAxes  FollAlignAxisA=+Z  BaseAlignAxisA=-X  FollAlignAxisB=+Y  BaseAlignAxisB=+Y  RotationStandardAxis=+Z  RotationAngle=0.0  RotationAngleUnits=deg  RotationArbitraryAxis=[0 0 1]  RotationSequenceAxes=FollowerAxes  RotationSequence=XYX  RotationSequenceAngles=[0 0 0]  RotationSequenceAnglesUnits=deg  RotationMatrix=[1 0 0; 0 1 0; 0 0 1]  Quaternion=[1 0 0 0]  TranslationMethod=None  TranslationCartesianOffset=[0 0 0]  TranslationCartesianOffsetUnits=m  TranslationStandardAxis=+Z  TranslationStandardOffset=0  TranslationStandardOffsetUnits=m  TranslationROffset=0  TranslationROffsetUnits=m  TranslationThetaOffset=0  TranslationThetaOffsetUnits=deg  TranslationZOffset=0  TranslationZOffsetUnits=m
  Transform S to B : sm_lib/Frames and Transforms/Rigid Transform  RotationMethod=AlignedAxes  FollAlignAxisA=+Z  BaseAlignAxisA=-Y  FollAlignAxisB=+X  BaseAlignAxisB=+X  RotationStandardAxis=+Z  RotationAngle=0.0  RotationAngleUnits=deg  RotationArbitraryAxis=[0 0 1]  RotationSequenceAxes=FollowerAxes  RotationSequence=XYX  RotationSequenceAngles=[0 0 0]  RotationSequenceAnglesUnits=deg  RotationMatrix=[1 0 0; 0 1 0; 0 0 1]  Quaternion=[1 0 0 0]  TranslationMethod=None  TranslationCartesianOffset=[0 0 0]  TranslationCartesianOffsetUnits=m  TranslationStandardAxis=+Z  TranslationStandardOffset=0  TranslationStandardOffsetUnits=m  TranslationROffset=0  TranslationROffsetUnits=m  TranslationThetaOffset=0  TranslationThetaOffsetUnits=deg  TranslationZOffset=0  TranslationZOffsetUnits=m
  Transform S to B 2 : sm_lib/Frames and Transforms/Rigid Transform  RotationMethod=AlignedAxes  FollAlignAxisA=+Z  BaseAlignAxisA=+X  FollAlignAxisB=+Y  BaseAlignAxisB=+Y  RotationStandardAxis=+Z  RotationAngle=0.0  RotationAngleUnits=deg  RotationArbitraryAxis=[0 0 1]  RotationSequenceAxes=FollowerAxes  RotationSequence=XYX  RotationSequenceAngles=[0 0 0]  RotationSequenceAnglesUnits=deg  RotationMatrix=[1 0 0; 0 1 0; 0 0 1]  Quaternion=[1 0 0 0]  TranslationMethod=None  TranslationCartesianOffset=[0 0 0]  TranslationCartesianOffsetUnits=m  TranslationStandardAxis=+Z  TranslationStandardOffset=0  TranslationStandardOffsetUnits=m  TranslationROffset=0  TranslationROffsetUnits=m  TranslationThetaOffset=0  TranslationThetaOffsetUnits=deg  TranslationZOffset=0  TranslationZOffsetUnits=m
  World Frame : sm_lib/Frames and Transforms/World Frame
  F : PMIOPort  Side=Right
  wires:
  Bus Element In/1 -> Simulink-PS Converter/1
  Bus Element In1/1 -> Simulink-PS Converter1/1
  Bus Element In2/1 -> Simulink-PS Converter2/1
  Bus Element In3/1 -> Simulink-PS Converter3/1
  Bus Element In4/1 -> Simulink-PS Converter4/1
  Bus Element In5/1 -> Simulink-PS Converter5/1
  Constant/1 -> Signal Specification2/1
  [zw] -> Simulink-PS Converter4/2
  [zv] -> Simulink-PS Converter2/2, Simulink-PS Converter1/2, Simulink-PS Converter/2
  [zw] -> Simulink-PS Converter5/2
  [zw] -> Simulink-PS Converter3/2
  Constant1/1 -> Signal Specification1/1
  [zb] -> Simulink-PS Converter4/3
  [zb] -> Simulink-PS Converter5/3
  [za] -> Simulink-PS Converter/3, Simulink-PS Converter2/3, Simulink-PS Converter1/3
  [zb] -> Simulink-PS Converter3/3
  Signal Specification2/1 -> [zv]
  Signal Specification1/1 -> [za]
  Signal Specification3/1 -> [zb]
  Signal Specification4/1 -> [zw]
  Constant3/1 -> Signal Specification3/1
  Constant2/1 -> Signal Specification4/1
  connections:
  Transform H to S/RConn1 -- Revolute Slope/LConn1
  Transform H to S/LConn1 -- Revolute Heading/RConn1
  Revolute Bank/RConn1 -- Transform Plane/LConn1
  Transform Plane/RConn1 -- F/RConn1
  Simulink-PS Converter1/RConn1 -- Cartesian Joint/LConn3
  Revolute Heading/LConn1 -- Cartesian Joint/RConn1
  Transform S to B/LConn1 -- Revolute Slope/RConn1
  Transform S to B 2/RConn1 -- Revolute Bank/LConn1
  Transform S to B/RConn1 -- Transform S to B 2/LConn1
  Simulink-PS Converter/RConn1 -- Cartesian Joint/LConn2
  Simulink-PS Converter4/RConn1 -- Revolute Slope/LConn2
  Cartesian Joint/LConn1 -- World Frame/RConn1
  Simulink-PS Converter3/RConn1 -- Revolute Heading/LConn2
  Simulink-PS Converter5/RConn1 -- Revolute Bank/LConn2
  Simulink-PS Converter2/RConn1 -- Cartesian Joint/LConn4

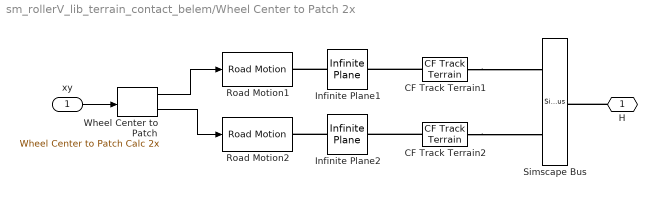
== system sm_rollerV_lib_terrain_contact_belem/Wheel Center to Patch 2x ==
  xy : Inport
  CF Track Terrain1 : sm_trackV_lib_terrain_contact_elem/CF Track Terrain  NormalStiffness=NormalStiffness  NormalDamping=NormalDamping  NormalTransitionRegionWidth=NormalTransitionRegionWidth  CoefficientOfDynamicFriction=CoefficientOfDynamicFriction  CoefficientOfStaticFriction=CoefficientOfStaticFriction  FrictionalCriticalVelocity=FrictionalCriticalVelocity
  CF Track Terrain2 : sm_trackV_lib_terrain_contact_elem/CF Track Terrain  NormalStiffness=NormalStiffness  NormalDamping=NormalDamping  NormalTransitionRegionWidth=NormalTransitionRegionWidth  CoefficientOfDynamicFriction=CoefficientOfDynamicFriction  CoefficientOfStaticFriction=CoefficientOfStaticFriction  FrictionalCriticalVelocity=FrictionalCriticalVelocity
  Infinite Plane1 : sm_lib/Curves and Surfaces/Infinite Plane  GraphicType=Rectangle  GraphicPlaneWidth=patch_x  GraphicPlaneWidthUnits=m  GraphicPlaneHeight=patch_y  GraphicPlaneHeightUnits=m  GraphicVisPropType=SimpleVisualProperties  GraphicDiffuseColor=patch_clr  GraphicOpacity=patch_opc  GraphicSpecularColor=[0.5 0.5 0.5 1.0]  GraphicAmbientColor=[0.15 0.15 0.15 1.0]  GraphicEmissiveColor=[0.0 0.0 0.0 1.0]  GraphicShininess=75
  Infinite Plane2 : sm_lib/Curves and Surfaces/Infinite Plane  GraphicType=Rectangle  GraphicPlaneWidth=patch_x  GraphicPlaneWidthUnits=m  GraphicPlaneHeight=patch_y  GraphicPlaneHeightUnits=m  GraphicVisPropType=SimpleVisualProperties  GraphicDiffuseColor=patch_clr  GraphicOpacity=patch_opc  GraphicSpecularColor=[0.5 0.5 0.5 1.0]  GraphicAmbientColor=[0.15 0.15 0.15 1.0]  GraphicEmissiveColor=[0.0 0.0 0.0 1.0]  GraphicShininess=75
  Road Motion1 : $bdroot/Road Motion
  Road Motion2 : $bdroot/Road Motion
  Simscape Bus : SimscapeBus  HierarchyStrings=S1;S2
  Wheel Center to Patch : $bdroot/Wheel Center to Patch Calc 2x  road_pz_x=road_pz_x  road_pz_z=road_pz_z  road_qy_x=road_qy_x  road_qy_qy=road_qy_qy  tfilter=tfilter
      settings: LibrarySourceBlock=|
      | sm_excv_uneven_road_lib/Patch Position
      | Rough Road1
  H : PMIOPort  Side=Right
  wires:
  xy/1 -> Wheel Center to Patch/1
  Wheel Center to Patch/2 -> Road Motion2/1
  Wheel Center to Patch/1 -> Road Motion1/1
  connections:
  Infinite Plane1/LConn1 -- Road Motion1/RConn1
  CF Track Terrain1/LConn1 -- Infinite Plane1/RConn1
  Infinite Plane2/LConn1 -- Road Motion2/RConn1
  CF Track Terrain2/LConn1 -- Infinite Plane2/RConn1
  H/RConn1 -- Simscape Bus/RConn1
  CF Track Terrain1/RConn1 -- Simscape Bus/LConn1
  CF Track Terrain2/RConn1 -- Simscape Bus/LConn2

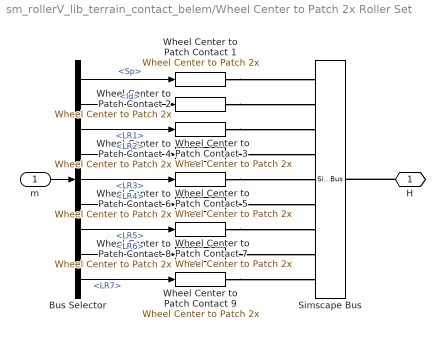
== system sm_rollerV_lib_terrain_contact_belem/Wheel Center to Patch 2x Roller Set ==
  m : Inport
  Bus Selector : BusSelector  OutputSignals=Underc.Sp,Underc.Id,Underc.LR1,Underc.LR2,Underc.LR3,Underc.LR4,Underc.LR5,Underc.LR6,Underc.LR7
  Simscape Bus : SimscapeBus  HierarchyStrings=L1;L2;L3;L4;L5;L6;L7;L8;L9
  Wheel Center to Patch Contact {1..9} (9 alike) : $bdroot/Wheel Center to Patch 2x  road_pz_x=road_pz_x  road_pz_z=road_pz_z  road_qy_x=road_qy_x  road_qy_qy=road_qy_qy  tfilter=tfilter  patch_clr=patch_clr  patch_opc=patch_opc  patch_x=patch_x  patch_y=patch_y  NormalStiffness=NormalStiffness  NormalDamping=NormalDamping  NormalTransitionRegionWidth=NormalTransitionRegionWidth  CoefficientOfDynamicFriction=CoefficientOfDynamicFriction  CoefficientOfStaticFriction=CoefficientOfStaticFriction  FrictionalCriticalVelocity=FrictionalCriticalVelocity
      settings: LibrarySourceBlock=sm_excv_uneven_road_lib/Rough Road 1 Roller1
  H : PMIOPort  Side=Right
  wires:
  Bus Selector/3 -> Wheel Center to Patch Contact 3/1  "<LR1>"
  Bus Selector/9 -> Wheel Center to Patch Contact 9/1  "<LR7>"
  Bus Selector/8 -> Wheel Center to Patch Contact 8/1  "<LR6>"
  Bus Selector/4 -> Wheel Center to Patch Contact 4/1  "<LR2>"
  Bus Selector/5 -> Wheel Center to Patch Contact 5/1  "<LR3>"
  Bus Selector/2 -> Wheel Center to Patch Contact 2/1  "<Id>"
  Bus Selector/7 -> Wheel Center to Patch Contact 7/1  "<LR5>"
  Bus Selector/6 -> Wheel Center to Patch Contact 6/1  "<LR4>"
  Bus Selector/1 -> Wheel Center to Patch Contact 1/1  "<Sp>"
  m/1 -> Bus Selector/1
  connections:
  Wheel Center to Patch Contact 8/RConn1 -- Simscape Bus/LConn8
  Wheel Center to Patch Contact 3/RConn1 -- Simscape Bus/LConn3
  Wheel Center to Patch Contact 7/RConn1 -- Simscape Bus/LConn7
  Wheel Center to Patch Contact 1/RConn1 -- Simscape Bus/LConn1
  Wheel Center to Patch Contact 6/RConn1 -- Simscape Bus/LConn6
  Wheel Center to Patch Contact 9/RConn1 -- Simscape Bus/LConn9
  Wheel Center to Patch Contact 2/RConn1 -- Simscape Bus/LConn2
  Wheel Center to Patch Contact 5/RConn1 -- Simscape Bus/LConn5
  Wheel Center to Patch Contact 4/RConn1 -- Simscape Bus/LConn4
  H/RConn1 -- Simscape Bus/RConn1

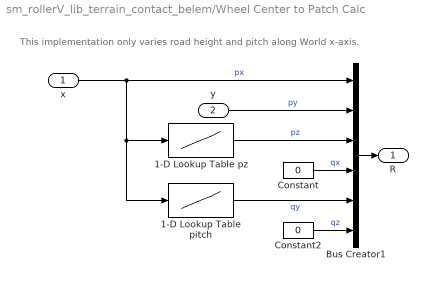
== system sm_rollerV_lib_terrain_contact_belem/Wheel Center to Patch Calc ==
  note: This implementation only varies road height and pitch along World x-axis.
  x : Inport
  y : Inport  Port=2
  1-D Lookup Table pitch : Lookup_n-D  NumberOfTableDimensions=1  BreakpointsForDimension1=road_qy_x  Table=road_qy_qy  InterpMethod=Akima spline  InternalRulePriority=Speed  RndMeth=Simplest
  1-D Lookup Table pz : Lookup_n-D  NumberOfTableDimensions=1  BreakpointsForDimension1=road_pz_x  Table=road_pz_z  InterpMethod=Akima spline  InternalRulePriority=Speed  RndMeth=Simplest
  Bus Creator1 : BusCreator  Inputs=6
  Constant : Constant  Value=0
  Constant2 : Constant  Value=0
  R : Outport
  wires:
  1-D Lookup Table pz/1 -> Bus Creator1/3  "pz"
  1-D Lookup Table pitch/1 -> Bus Creator1/5  "qy"
  Bus Creator1/1 -> R/1
  Constant2/1 -> Bus Creator1/6  "qz"
  Constant/1 -> Bus Creator1/4  "qx"
  y/1 -> Bus Creator1/2  "py"
  x/1 -> 1-D Lookup Table pitch/1, 1-D Lookup Table pz/1, Bus Creator1/1  "px"

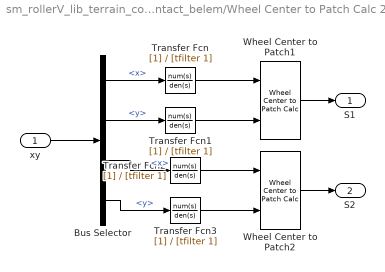
== system sm_rollerV_lib_terrain_contact_belem/Wheel Center to Patch Calc 2x ==
  xy : Inport
  Bus Selector : BusSelector  OutputSignals=S1.x,S1.y,S2.x,S2.y
  Transfer Fcn{,1..3} (4 alike) : TransferFcn  Denominator=[tfilter 1]
  Wheel Center to Patch1 : $bdroot/Wheel Center to Patch Calc  road_pz_x=road_pz_x  road_pz_z=road_pz_z  road_qy_x=road_qy_x  road_qy_qy=road_qy_qy
      settings: LibrarySourceBlock=sm_excv_uneven_road_lib/Rough Road Calc1
  Wheel Center to Patch2 : $bdroot/Wheel Center to Patch Calc  road_pz_x=road_pz_x  road_pz_z=road_pz_z  road_qy_x=road_qy_x  road_qy_qy=road_qy_qy
      settings: LibrarySourceBlock=sm_excv_uneven_road_lib/Rough Road Calc1
  S1 : Outport
  S2 : Outport  Port=2
  wires:
  Bus Selector/2 -> Transfer Fcn1/1  "<y>"
  Bus Selector/1 -> Transfer Fcn/1  "<x>"
  xy/1 -> Bus Selector/1
  Wheel Center to Patch1/1 -> S1/1
  Wheel Center to Patch2/1 -> S2/1
  Bus Selector/3 -> Transfer Fcn2/1  "<x>"
  Bus Selector/4 -> Transfer Fcn3/1  "<y>"
  Transfer Fcn/1 -> Wheel Center to Patch1/1
  Transfer Fcn1/1 -> Wheel Center to Patch1/2
  Transfer Fcn2/1 -> Wheel Center to Patch2/1
  Transfer Fcn3/1 -> Wheel Center to Patch2/2
